simulink model "Lab4_DataLog_hw_solution"  (R2025b)
settings: Solver=FixedStepDiscrete  StartTime=0.0  StopTime=30  FixedStep=50e-6  RelTol=1e-3  EnableMultiTasking=on
undefined symbols (not defined in the file or in its folder): A0, A4, ADC, B0, C10, C11, C12, C13, C14, C15, C2, C3, C4, C5, CND4max, D0, D1, D10, D12, D13, D14, D2, D3, D4, D5, D6, D9, DiscIntNeverNeededParam, Max, MaxPer, ms, NumBits1, NumBits2, P1, P17, P20, P35, P36, P37, P38, P43, P44, P45, P46, P47, P48, P49, P50, P51, P52, P54, P55, P58, P59, P61, P62, P63, Pin, PWM1_Trg1, Resol ... (+2)
libraries: simulink x31, MCHP_Blockset x20
(part 1 of 5)
PreSaveFcn:
  | try, MCHP_Fun.syncToolchainOptions(gcs); catch, end  %MCHP_PRESAVE_SYNC_V1
Description:
  | v1.0 (2026-06-12): created template from Developpements dev model; added Title/HowTo root annotations + inner PINOUT (Pegasus pin map), fixed stale MaskType (CK256MP508->AK512MC510), SimulationMode external->normal.
  | v1.1 (2026-06-12): fancy annotation pass - coloured header band, spec badges, boxed callouts, keyboard-key HowTo, category-coloured PINOUT.
  | v1.1 (2026-06-12): fancy annotation pass - coloured header band, spec badges, boxed callouts, keyboard-key HowTo, category-coloured PINOUT.
  | v1.2 (2026-06-13): folded original detailed pinout into the new PINOUT (added System/Master/Compiler, PWM-config, UART-baud, Digital-I/O sections); removed superseded <!DOCTYPE> pinout (had M1_LED2=RA5 error) and old UART note; deduplicated PINOUT. Kept diagram-area section labels.
settings Model: SimulationMode=external  ExtModeEnableFloating=off  ExtModeTrigDuration=20  Creator=Lubin Kerhuel  LastModifiedBy=Lubin Kerhuel
settings SolverCC: AlgebraicLoopSolver=TrustRegion
settings OptimizationCC: DefaultUnderspecifiedDataType=single  EnhancedBackFolding=on  BooleansAsBitfields=on  PassReuseOutputArgsAs=Individual arguments  ZeroExternalMemoryAtStartup=off  ZeroInternalMemoryAtStartup=off  OptimizeBlockOrder=speed  DifferentSizesBufferReuse=on  EfficientTunableParamExpr=on
settings DebuggingCC: MultiTaskDSMMsg=none  MultiTaskCondExecSysMsg=none  MultiTaskRateTransMsg=warning  ParameterTunabilityLossMsg=error  ArithmeticOperatorsInVariantConditions=warning
settings HardwareCC: ProdBitPerPointer=32.0  ProdBitPerSizeT=32.0  ProdBitPerPtrDiffT=32.0  ProdLargestAtomicInteger=Long  ProdWordSize=32.0  ProdLongLongMode=on  ProdHWDeviceType=Generic->Custom
settings ModelReferenceCC: ModelReferenceNumInstancesAllowed=Single
settings SFSimCC: MATLABDynamicMemAlloc=off  CustomCodeUndefinedFunction=UseInterfaceOnly
settings RTWCC: SystemTargetFile=MCHP_dsPIC33A_noTMF_stf.tlc  TLCOptions="-aExtModeXCPClassicInterface=0  -aCreateExtModeTypes=1 -aExtModeXCPSimulationTimeInTicks=1"  TemplateMakefile=MCHP_dsPIC33A.tmf  Toolchain=MPLAB XC-DSC - v4.00 for dsPIC DSCs (Microchip)  BuildConfiguration=Specify  GPUComputeCapability=3.5  Description=Microchip Embedded Target dsPIC33A no TMF (real-time)
settings CodeAppCC: ForceParamTrailComments=on  IgnoreCustomStorageClasses=off  MaxIdLength=255.0  OperatorAnnotations=on  SimulinkDataObjDesc=on  SFDataObjDesc=on  InsertBlockDesc=on
settings STFCustomTargetCC: SystemTargetFile=MCHP_dsPIC33A_noTMF_stf.tlc  TargetLangStandard=C99 (ISO)  CodeReplacementLibrary=Microchip Code Replacement Library for dsPIC33A - (experimental)  MultiwordLength=256.0  ConcurrentExecutionCompliant=off  CombineOutputUpdateFcns=on  CombineSignalStateStructs=on  ERTCustomFileBanners=on  SubcomponentCodeInterfacePackaging=Nonreusable function  RemoveResetFunc=on  MATLABClassNameForMDSCustomization=Simulink.SoftwareTarget.ERTCustomization  GRTInterface=off  UseToolchainInfoCompliant=on  TIMER_PRESCALER="[-1 -1 -1  0  0 -1 -1 -1 -1 -1 -1 -1]"  GCC1=xc-dsc-gcc.exe  MCHP_MULTITHREAD_COMPILATION=on  LDFLAGS='--heap=1024,--report-mem,-Map=$(PRODUCT_NAME).map,-cref,-lq-dsp,--memorysummary,memoryfile.xml,--gc-sections'  ProduceHexOutput=off  MCHP_AUTO_FLASH=off  HOST_PLATFORM=PC  GCCPATH=C:/PROGRA~1/MICROC~1/xc-dsc/v4.00/bin  RTWGenSettings_txt="s.RefMasterBlk='Lab4_DataLog_hw_solution/BOARD MCLV-48V-300W dsPIC33AK512MC510 MC DIM1/Microchip Master';s.ChipIdN='[33  512  510]';s.ChipIdL1='AK';s.ChipIdL2='MC';s.ChipIdL3=' ';s.arch3='33A';s.ChipId='33AK512MC510';s.Arch='8';s.bitFieldsSFR='7';s.ChipRAM='32768';s.ChipRAM_XBegin='16384';s.ChipRAM_dma='[-1 -1]';s.AIVT_EN='0';s.FuseConfigTxt='#pragma config FICD_JTAGEN = OFF\\\\n#pragma config FWDT_WDTEN = SW\\\\n  ';s.TimeStep_Timer='-1';s.TimeStep_SyncADC='1';s.ADPCFG='0';s.ANSEL_Exist='1';s.ANSEL='[61439     -1  13287  40832      1     -1     -1     -1     -1     -1     -1]';s.TRIS='[65535  65535  65511  65520  65523  65533     -1     -1     -1     -1     -1     -1     -1     -1     -1     -1     -1     -1     -1     -1     -1     -1     -1     -1     -1     -1     -1     -1     -1     -1     -1     -1     -1     -1     -1     -1     -1     -1     -1     -1     -1     -1     -1     -1     -1     -1     -1     -1     -1     -1     -1     -1     -1     -1     -1     -1     -1]';s.RPOR='[-1         -1         -1         -1         -1         -1         -1         -1   83886080          6  352321536  318767104   33620995         -1         -1         -1         -1         -1         -1         -1         -1         -1         -1         -1         -1         -1         -1         -1         -1         -1         -1         -1         -1         -1         -1         -1]';s.RPINR='[-1       -1       -1       -1       -1       -1       -1       -1       -1    15935       -1       -1       -1  2818095       -1       -1       -1       -1       -1       -1       -1       -1       -1       -1       -1       -1       -1       -1]';s.LATSET='[-1 -1 -1 -1 -1 -1 -1 -1 -1 -1 -1 -1 -1 -1 -1 -1 -1 -1 -1 -1 -1 -1 -1 -1 -1 -1 -1 -1 -1 -1 -1 -1 -1 -1 -1 -1 -1 -1 -1 -1 -1 -1 -1 -1 -1 -1 -1 -1 -1 -1 -1 -1 -1 -1 -1 -1 -1]';s.LATCLR='[-1 -1 -1 -1 -1 -1 -1 -1 -1 -1 -1 -1 -1 -1 -1 -1 -1 -1 -1 -1 -1 -1 -1 -1 -1 -1 -1 -1 -1 -1 -1 -1 -1 -1 -1 -1 -1 -1 -1 -1 -1 -1 -1 -1 -1 -1 -1 -1 -1 -1 -1 -1 -1 -1 -1 -1 -1]';s.ODC='[-1 -1 -1 -1 -1 -1 -1 -1 -1 -1 -1 -1 -1 -1 -1 -1 -1 -1 -1 -1 -1 -1 -1 -1 -1 -1 -1 -1 -1 -1 -1 -1 -1 -1 -1 -1 -1 -1 -1 -1 -1 -1 -1 -1 -1 -1 -1 -1 -1 -1 -1 -1 -1 -1 -1 -1 -1]';s.CNPU='[-1 -1 -1 -1 -1 -1 -1 -1 -1 -1 -1 -1 -1 -1 -1 -1 -1 -1 -1 -1 -1 -1 -1 -1 -1 -1 -1 -1 -1 -1 -1 -1 -1 -1 -1 -1 -1 -1 -1 -1 -1 -1 -1 -1 -1 -1 -1 -1 -1 -1 -1 -1 -1 -1 -1 -1 -1]';s.CNPD='[-1 -1 -1 -1 -1 -1 -1 -1 -1 -1 -1 -1 -1 -1 -1 -1 -1 -1 -1 -1 -1 -1 -1 -1 -1 -1 -1 -1 -1 -1 -1 -1 -1 -1 -1 -1 -1 -1 -1 -1 -1 -1 -1 -1 -1 -1 -1 -1 -1 -1 -1 -1 -1 -1 -1 -1 -1]';s.PortConfigTxt=' ';s.CLKDIV='0';s.PLLFBD='-1';s.PLLDIV='16815713';s.QUARTZ='8000000';s.SWITCH_OSC='16386';s.PLLRNG='-1';s.MASTER_BusyFlag='-1';s.POWERSAVE='0';s.MIPS='200000000';s.FLASH_ECC='0';s.PBxDIV='[-1]';s.CLKx_INTDIV='[-1 -1 -1 -1  0  1  0  0  0 -1 -1  0  0]';s.CLKx_FRACDIV='[-1   -1   -1   -1    0  256    0    0    0   -1   -1    0    0]';s.AN_type2='1';s.ACLKCON_reg='-1';s.FRC_TUN_REG='0';s.BFRC_TUN_REG='0';s.nTIMERS='3';s.nSCCP='9';s.DOS_04094_cpu_33a_v1_dspic33a='1';s.DOS_04436_perseus_dspic33a='0';s.DOS_04928_gpio_ports_upb_v2_dspic33a='1';s.DOS_02672_math_progcrc_upb_v1_dspic33a='1';s.DOS_04993_sec_32bit_cp_upb_v1_dspic33a='1';s.DOS_03459_adc_pc_ctrl_upb_v2_dspic33a='0';s.DOS_04302_pwm_pc_upb_v3_dspic33a='0';s.DOS_03076_uart_protocol_upb_v1_dspic33a='1';s.DOS_01482_spi_i2s_upb_v1_dspic33a='1';s.DOS_05155_i2c_upb_v4_dspic33a='1';s.DOS_02359_sent_j2716_upb_v1_dspic33a='1';s.DOS_05177_qei_32b_upb_v2_dspic33a='1';s.DOS_01512_ccp_mccp_upb_v1_dspic33a='1';s.DOS_03496_dac_pdm_nbit_upb_v2_dspic33a='0';s.DOS_02673_tmr_classa_upb_v1_dspic33a='1';s.DOS_04776_perf_mon_upb_v1_dspic33a='1';s.DOS_03680_pfm_pbu_33a_upb_v1_dspic33a='1';s.DOS_04649_sec_pac_upb_v0_dspic33a='0';s.DOS_03966_io_integrity_monitor_upb_v1_dspic33a='1';s.DOS_04641_biss_master_upb_v1_dspic33a='1';s.DOS_04077_dma_upb_v1_dspic33a='1';s.DOS_04549_nvm_ctrl_32bit_upb_v1_dspic33a='1';s.DOS_04449_clk_cru_33a_upb_v1_dspic33a='1';s.DOS_03850_clk_monitor_upb_v1_dspic33a='1';s.DOS_04342_osc_rc8mhz_ctrl_upb_v4_dspic33a='1';s.DOS_04650_wdt_upb_v4_dspic33a='1';s.DOS_05178_ptg_pc_upb_v2_dspic33a='1';s.DOS_04181_data_ram_ctrl_upb_v1_dspic33a='1';s.DOS_04735_wdt_dmt_upb_v6_dspic33a='1';s.DOS_01577_cla_clc_upb_v1_dspic33a='1';s.DOS_03516_pwr_sib_upb_v3_dspic33a='0';s.DOS_03495_amp_pad_opamp_ctrl_upb_v2_dspic33a='1';s.DOS_02481_WACK_MC_Config='0';s.DOS_03088_pfm_cache_ocp_v2_WACK='0';s.DOS_02819_pfm_ctrl_32bit_upb_v2='0';s.DOS_02674_wdt_upb_v1_32bit='0';s.DOS_01520_wdt_dmt_upb_v1='0';s.DOS_02869_icd_jtag_bvci_upb_v2='0';s.DOS_02823_WACJ_clk_cru_upb_v2='0';s.DOS_02823_WACN_clk_cru_upb_v2='0';s.DOS_01423_RPINRx='0';s.DOS_02481_RPORx='0';s.DOS_02511_pwr_sib_upb_v1_32bit='0';s.DOS_02907_WACN_GP_int_evic_v3='0';s.DOS_01500_dma_bvci_v2='0';s.DOS_02141_tmr_classa_pb_v2='0';s.DOS_02815_tmr_classb_upb_v1='0';s.DOS_00740_icap_pb_v1='0';s.DOS_00749_ocmp_pb_v1='0';s.DOS_01441_i2c_upb_v1_32bit='0';s.DOS_01329_spi_pb_v2='0';s.DOS_02478_uart_irda_upb_v1_32bit='0';s.DOS_03554_cmp_control_upb_v2_32bit='0';s.DOS_01445_dac_nbit__control_upb_v1_32bit='0';s.DOS_01461_afe_ctmu_con_upb_v1='0';s.DOS_01577_cla_clc_upb_v1_32bit='0';s.DOS_02467_gpio_ports_upb_v1='0';s.DOS_02508_adc_sar_ctrl_upb_v1_PIC32MK='0';s.DOS_01261_tmr_rtcc_pb_v2='0';s.DOS_01475_lpwr_deep_sleep_ctrl_v2='0';s.DOS_EIP_00136_ssx_v1='0';s.DOS_02907_WACK_MC_int_evic_v3='0';s.DOS_02514_dfm_strl_sst_upb_v1='0';s.DOS_02472_ppi_pmp16_upb_v1='0';s.DOS_02813a_usb_otgcore_pb_v3='0';s.DOS_02481_WACP_Config='0';s.DOS_02907_WACP_int_evic_v3='0';s.DOS_01477_pwm_mc_upb_v1='0';s.DOS_01494_qei_32b_upb_v1='0';s.DOS_02508_WACP_adc_sar_ctrl_upb_v1='0';s.DOS_01261_tmr_rtcc_WACJ_K_N_P_pb_v2='0';s.DOS_02907_WACN_MC_int_evic_v3='0';s.DOS_03247_can_fd_upb_v2_pic32mk='0';s.DOS_02481_WACJ_MC_Config='0';s.DOS_02569_pfm_cache_ocp_v1='0';s.DOS_02481_WACJ_MC_int_evic_v3='0';s.DOS_01459_ptg_pc_upb_v1_SIC='0';s.DOS_01427_cmp_control_upb_v1_32bit='0';s.DOS_01152_can_bvci_v1='0';s.DOS_02787_WACD_Config='0';s.DOS_00800_dac_4bit_ctrl_pb_v1='0';s.DOS_01539_icd_jtag_pb_v2='0';s.DOS_02823_clk_cru_upb_v2='0';s.DOS_01423_RPORx='0';s.DOS_02907_WACD_int_evic_v3='0';s.DOS_00734_uart_irda_pb_v1='0';s.DOS_00687_tmr_classa_pb_v1='0';s.DOS_00745_tmr_classb_pb_v1='0';s.DOS_02508_adc_sar_ctrl_upb_v1='0';s.DOS_00866_cmp_control_pb_v2='0';s.DOS_01114_eth_bvci_v1='0';s.DOS_02831_usb_clk_rst_v2='0';s.DOS_01643_pfm_cache_ahb_v2='0';s.DOS_EIP_00206r5_sqi_v2='0';s.DOS_EIP_00124_usb_hs_otgcore_v1='0';s.DOS_EIP_00218_math_rng_ahbs_v2='0';s.DOS_EIP_00109_ebi_v1='0';s.DOS_EIP_00158_crypto_v1='0';s.DOS_05557_serpens_dspic33a='0';s.DOS_05972_adc_12b_upb_v3_adc_dspic33a='0';s.DOS_03681_bmx_33a_upb_v1_dspic33a='0';s.DOS_05226_pwm_pc_upb_v4_dspic33a='1';s.DOS_05514_qei_32b_upb_v3_dspic33a='0';s.DOS_02050_tmr_rtcc_upb_v1_dspic33a='0';s.DOS_05431_dac_pdm_nbit_upb_v3_dspic33a='1';s.DOS_04649_sec_pac_upb_serpens_dspic33a='0';s.DOS_05801_dma_upb_v2_dspic33a='0';s.DOS_05692_pwr_sib_upb_v5_dspic33a='0';s.DOS_05420_amp_vref_ctl_upb_v1_dspic33a='1';s.DOS_05346_sec_cam_v2_dspic33a='1';s.DOS_06006_adc_soft_code_seq_v2_adc_dspic33a='0';s.DOS_05442_icd_trace_33a_v1_dspic33a='0';s.DOS_04537_can_fd_upb_v3_dspic33a='1';s.DOS_05308_pegasus_dspic33a='1';s.DOS_02976_adc_12b_upb_v2_dspic33a='1';s.DOS_05404_adc_pc_ctrl_upb_v3_dspic33a='1';s.DOS_05226_apwm_pc_upb_v4_dspic33a='1';s.DOS_04649_sec_pac_upb_v1_dspic33a='1';s.DOS_05461_pwr_sib_upb_v4_dspic33a='1';s.DOS_03267_adc_soft_code_seq_v1_dspic33a='1';s.DOS_05830_blueRidge_dspic33a='0';s.DOS_05972_adc_12b_upb_v3_itc_dspic33a='0';s.DOS_05828_pfm_pbu_33a_upb_v2_dspic33a='0';s.DOS_05765_math_rdc_upb_v1_32bit='0';s.DOS_05908_math_cic_upb_v2_32bit='0';s.DOS_05592_pwr_monitor_sib_upb_v1='0';s.DOS_05924_bus_dual_die_upb_v2='0';s.DOS_06048_sec_cam_v3_dspic33a='0';s.DOS_05922_i3c_upb_v1_32bit='0';s.DOS_06006_adc_soft_code_seq_v2_dspic33a='0';s.DOS_02551_cpu_16bit_v7='0';s.DOS_01520_wdt_dmt_upb_v1_16bit='0';s.DOS_02359a_sent_j2716_upb_v1='0';s.DOS_02672_math_progcrc_upb_v1_16bit='0';s.DOS_01577_cla_clc_upb_v1='0';s.DOS_02915_ecc_v2='0';s.DOS_02673_tmr_classa_upb_v1_16bit='0';s.DOS_01494_qei_32b_upb_v1_16bit='0';s.DOS_01441_i2c_upb_v1_16bit_TLAH='0';s.DOS_03076_uart_protocol_upb_v1_16bit='0';s.DOS_01482='0';s.DOS_01483_pwm_16bit='0';s.DOS_04884_WAC0B='0';s.DOS_02316_nvm_ctrl_v1_16bit='0';s.DOS_03349_amp_pad_opamp_ctrl_upb_v1='0';s.DOS_02653_afe_current_bias_ctrl_upb_v1_16bit='0';s.DOS_01459_ptg_pc_upb_v1_16bit='0';s.DOS_01512_ccp_mccp_upb_v1_16bit='0';s.DOS_02519_dma_sfr_16bit_v2='0';s.DOS_02508c11='0';s.DOS_02475_dac_pdm_nbit_upb_v1_16bit='0';s.DOS_02467_gpio_upb_v1_16bit='0';s.DOS_00805_rst_integration_v4='0';s.DOS_02659_clk_sib_v12='0';s.DOS_02237_osc_dco_ctrl_upb_v1_16bit='0';s.DOS_02674_wdt_upb_v1_16bit='0';s.DOS_01407='0';s.DOS_03247_CAN_FD_UPB_V2_16_bit='0';s.DOS_03994_WAC07='0';s.DOS_02472_ppi_pmp16_upb_v1_16bit='0';s.DOS_02949_WACG='0';s.DOS_02552_msi_upb_v1_Master='0';s.DOS_03667_pwm_pc_upb_v2_16bit='0';s.DOS_04180_drm_ctrl_ecc_v1='0';s.DOS_03431_STX03='0';s.DOS_03516_pwr_sib_upb_v3='0';s.DOS_02552_msi_upb_v1_Slave='0';s.DOS_04621_amp_pga_ctrl_upb_v3='0';s.DOS_02497_WACV='0';s.DOS_02593_amp_pga_ctrl_pb_v2_16bit='0';s.DOS_03029_WACH='0';s.DOS_01483_apwm_16bit='0';s.DOS_04797_WAC0A='0';s.DOS_04797_WAC09='0';s.DOS_03662_WACU='0';s.DOS_00794='0';s.DOS_00931='0';s.DOS_00932='0';s.DOS_00942='0';s.DOS_00938='0';s.DOS_00996='0';s.DOS_00997='0';s.DOS_00998='0';s.DOS_00209='0';s.DOS_01555_adc='0';s.DOS_01293='0';s.DOS_00828='0';s.DOS_01116='0';s.DOS_01017_RPORx='0';s.DOS_01017_RPINRx='0';s.DOS_01555_nvm_tsmc18_v2_16bit='0';s.DOS_00804='0';s.DOS_00826='0';s.DOS_01555_TLAK_PMDx='0';s.DOS_01555_TLAK_INT_='0';s.DOS_00933='0';s.DOS_01555='0';s.DOS_01555_ptg='0';s.DOS_00929='0';s.DOS_00958='0';s.DOS_01117_PORTx='0';s.DOS_00999='0';s.DOS_01198='0';s.DOS_01041='0';s.DOS_00892='0';s.DOS_01287_TLAC_PMDx='0';s.DOS_01287_TLAC_INT_='0';s.DOS_01424='0';s.DOS_01332='0';s.DOS_01113='0';s.DOS_01017_PMDx='0';s.DOS_00927='0';s.DOS_01080='0';s.DOS_01468_PMBA_current_source='0';s.DOS_02291_PGA='0';s.DOS_01467_Comparator='0';s.DOS_01498_TLAY='0';s.DOS_00993_PLL_120MHz='0';s.DOS_01332_ptg_pc_v1='0';s.DOS_00958_pwm_TLAY='0';s.TLAY_IOPorts='0';s.DOS_00929q='0';s.DOS_02415_spi_v5='0';s.DOS_RPINRx_16bit_2='0';s.DOS_01497_TLAH_PMDx='0';s.DOS_02550_TLAL_INT='0';s.DOS_00958_pwm_TLAH='0';s.DOS_01287_TLAH_INT_='0';s.DOS_00794_cpu_16bit_v3='0';s.DOS_02192_TLCD_PMDx='0';s.DOS_02192_TLCD_INT_='0';s.DOS_02192_cmp='0';s.DOS_00958_pwm_TLCD='0';s.DOS_02192_PORTx_TLCD='0';s.DOS_00936='0';s.DOS_00995='0';s.DOS_00546='0';s.DOS_00474='0';s.UART_TX_IMPLEMENTATION='[5  5]';s.UART_RX_IMPLEMENTATION='[6  6]';s.UART_TX_DMACHANNEL='[0  1]';s.UART_HALF_DUPLEX_MODE='[0  0]';s.UART_TX_THREAD_PROTECTION='[9  9]';"  TIMER_START="[0  0  0  1  0]"  OPTIM_GCC=-O3 -mno-eds-warn -mconst-in-data -mlarge-code -mlarge-data -mlarge-scalar -g -Wa,--reorder -ffunction-sections -fdata-sections  TIMER_WIDTH="[16  16  16  32  16  16  16  16  16  16  16  16]"  MCHP_CompiledTime_ModelSampleTimes_Txt=s(1).Value=reshape([0 0],1,2);s(1).Description='Continuous';s(1).ColorRGBValue=reshape([0 0 0],1,3);s(1).Annotation='Cont';s(1).TID=0;s(1).Owner=[];s(1).ComponentSampleTimes=[];s(2).Value=reshape([5e-05 0],1,2);s(2).Description='Discrete 1';s(2).ColorRGBValue=reshape(MCHP_Fun.Hex2num('[3FCF1F1F1F1F1F1F 3FC3131313131313 3FE5151515151515]'),1,3);s(2).Annotation='D1';s(2).TID=1;s(2).Owner=[];s(2).ComponentSampleTimes=[];s(3).Value=reshape([0.0001 0],1,2);s(3).Description='Discrete 2';s(3).ColorRGBValue=reshape(MCHP_Fun.Hex2num('[3FD0D0D0D0D0D0D1 3FD9D9D9D9D9D9DA 3FEFBFBFBFBFBFC0]'),1,3);s(3).Annotation='D2';s(3).TID=2;s(3).Owner=[];s(3).ComponentSampleTimes=[];s(4).Value=reshape([0.0005 0],1,2);s(4).Description='Discrete 3';s(4).ColorRGBValue=reshape(MCHP_Fun.Hex2num('[3FBC1C1C1C1C1C1C 3FE5555555555555 3FEBFBFBFBFBFBFC]'),1,3);s(4).Annotation='D3';s(4).TID=3;s(4).Owner=[];s(4).ComponentSampleTimes=[];s(5).Value=reshape([0.001 0],1,2);s(5).Description='Discrete 4';s(5).ColorRGBValue=reshape(MCHP_Fun.Hex2num('[3FD2121212121212 3FE9797979797979 3FE0D0D0D0D0D0D1]'),1,3);s(5).Annotation='D4';s(5).TID=4;s(5).Owner=[];s(5).ComponentSampleTimes=[];s(6).Value=reshape([0.01 0],1,2);s(6).Description='Discrete 5';s(6).ColorRGBValue=reshape(MCHP_Fun.Hex2num('[3FED5D5D5D5D5D5D 3FE7575757575757 3FC8181818181818]'),1,3);s(6).Annotation='D5';s(6).TID=5;s(6).Owner=[];s(6).ComponentSampleTimes=[];s(7).Value=reshape([0.1 0],1,2);s(7).Description='Discrete 6';s(7).ColorRGBValue=reshape(MCHP_Fun.Hex2num('[3FEF3F3F3F3F3F3F 3FEF7F7F7F7F7F7F 3FB5151515151515]'),1,3);s(7).Annotation='D6';s(7).TID=6;s(7).Owner=[];s(7).ComponentSampleTimes=[];s(8).Value=reshape([-1 -2],1,2);s(8).Description='Asynchronous 1';s(8).ColorRGBValue=reshape(MCHP_Fun.Hex2num('[3FE8181818181818 3FD7171717171717 3FEF7F7F7F7F7F7F]'),1,3);s(8).Annotation='A1';s(8).TID=7;s(8).Owner={ 'MCHP_MCLV48V300W_dsPIC33AK512MC510_DIM_HallSensors_DataLog/Interrupt'};s(8).ComponentSampleTimes=[];s(9).Value=reshape([Inf Inf],1,2);s(9).Description='Constant';s(9).ColorRGBValue=reshape(MCHP_Fun.Hex2num('[3FEA3A3A3A3A3A3A 3F90101010101010 3FE1717171717171]'),1,3);s(9).Annotation='Inf';s(9).TID=-2;s(9).Owner=[];s(9).ComponentSampleTimes=[];s(10).Value=[];s(10).Description='Multirate';s(10).ColorRGBValue=reshape(MCHP_Fun.Hex2num('[3FE1717171717171 3FD999999999999A 3F98181818181818]'),1,3);s(10).Annotation='M';s(10).TID=[];s(10).Owner=[];s(10).ComponentSampleTimes=[];  BIN2HEX=xc-dsc-bin2hex  TIMER_PERIOD="[0          0          0  199999999      65535]"  LINKER_SCRIPT=p33AK512MC510.gld  EXTMODE_DATA_UPLOAD=on  MCHP_XCP_MemoryBlockParameters=[10 10]  AssemblyListing=off  OBJDUMP=xc-dsc-objdump  AR1=xc-dsc-ar  LinkWithMaster=off  PIC_REF=33AK512MC510
settings ERTTargetCC: ExtMode=on  ExtModeTransport=1.0  ExtModeStaticAlloc=on  ExtModeStaticAllocSize=2048.0  ExtModeMexFile=ext_xcp  ExtModeMexArgs=1 34 8000000 './MCHP_MCLV48V300W_dsPIC33AK512MC510_DIM_HallSensors_DataLog.X/MCHP_MCLV48V300W_dsPIC33AK512MC510_DIM_HallSensors_DataLog.elf'  ExtModeIntrfLevel=Level2 - Open  InlinedParameterPlacement=Hierarchical  ERTSrcFileBannerTemplate=MCHP_dsPIC_code_template.cgt  ERTHdrFileBannerTemplate=MCHP_dsPIC_code_template.cgt  ERTDataSrcFileTemplate=MCHP_dsPIC_code_template.cgt  ERTDataHdrFileTemplate=MCHP_dsPIC_code_template.cgt  ERTCustomFileTemplate=MCHP_main.tlc  MaxLineWidth=110.0  DynamicArrayContainerType=coder::array  TargetLangStandard=C99 (ISO)  CodeReplacementLibrary=Microchip Code Replacement Library for dsPIC33A - (experimental)  ParMdlRefBuildCompliant=off  CompOptLevelCompliant=off  ConcurrentExecutionCompliant=off  CombineSignalStateStructs=on  SubcomponentCodeInterfacePackaging=Nonreusable function  SupportContinuousTime=on  SupportNonInlinedSFcns=on  ModelStepFunctionPrototypeControlCompliant=off  CPPClassGenCompliant=off

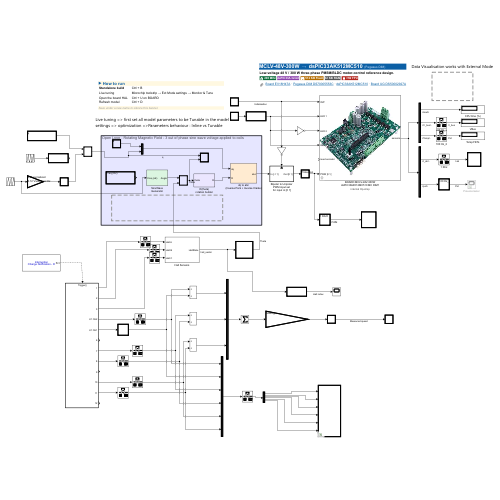
[thumbnail: Simulink's stored preview of the top-level diagram]
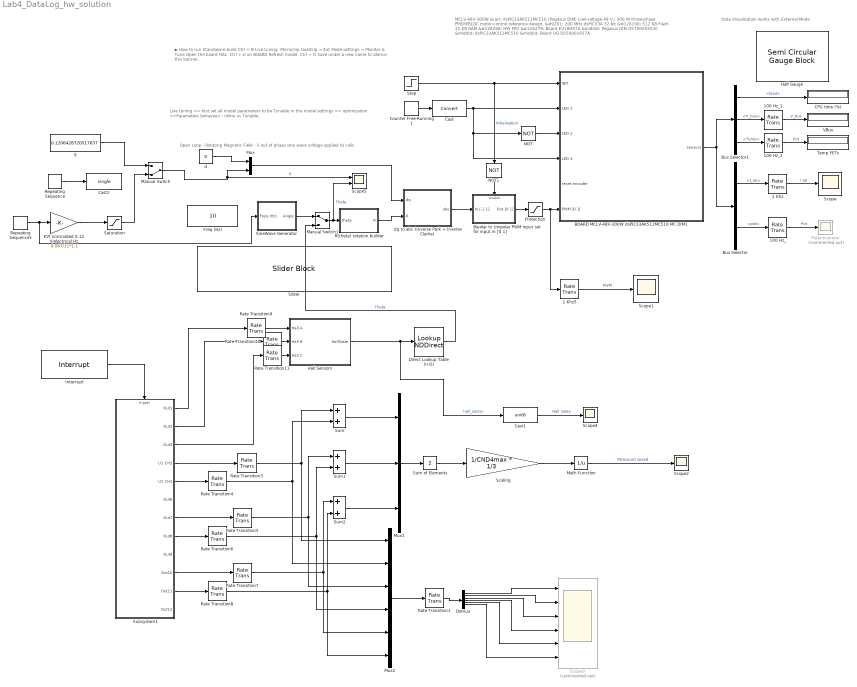
== system Lab4_DataLog_hw_solution ==
  note: Data Visualisation works with External Mode
  note: Open Loop - Rotating Magnetic Field - 3 out of phase sine wave voltage applied to coils
  note: MCLV-48V-300W &rarr; dsPIC33AK512MC510 (Pegasus DIM)
      | Low-voltage 48 V / 300 W three-phase PMSM/BLDC motor-control reference design.
      | &#9201; 200 MHz dsPIC33A 32-bit &#128190; 512 KB Flash 32 KB RAM &#128268; HW FPU
      | &#128279; Board EV18H47A &middot; Pegasus DIM DS70005553C &middot; dsPIC33AK512MC510 &middot; Board UG DS50002927A
  note: ▶ How to run
      | Standalone build
      |
      | Ctrl + B
      |
      | Live tuning
      | ​
      | Microchip toolstrip → Ext Mode settings → Monitor & Tune
      |
      | Open the board HAL
      | ​
      | Ctrl + U on BOARD
      |
      | Refresh model
      | ​
      | Ctrl + D
      |
      | Save under a new name to silence this banner.
  note: Live tuning => first set all model parameters to be Tunable in the model settings => optimization =>Parameters behaviour : Inline vs Tunable
  1 Khz : RateTransition  Deterministic=off  OutPortSampleTime=50e-6
  1 Khz5 : RateTransition  Deterministic=off  OutPortSampleTime=.001
  100 Hz_ : RateTransition  Deterministic=off  OutPortSampleTime=.01
  100 Hz_1 : RateTransition  Deterministic=off  OutPortSampleTime=.01
  100 Hz_2 : RateTransition  Deterministic=off  OutPortSampleTime=.01
  BOARD MCLV-48V-300W dsPIC33AK512MC510 MC DIM1 : Subsystem  mask(MCLV-48V-300W - dsPIC33AK512MC510 MC DIM){boardVariants=internal Op-Amp, n=4, QEIResolution=1000, QEI_Reset=on logical input (software), QEI_Offset_settings=0, QEIOffset=0}
      mask prompts: boardVariants "board variants"; n "Motor poles pairs"; QEIResolution "Optical encoder resolution per mechanical rotation (lines)"; QEI_Reset "Optical encoder reset"; QEI_Offset_settings "Optical encoder offset (mechanical in rad)"; QEIOffset "Optical encoder offset (mechanical in rad)"
      mask help:
      | Template for motor control algorithm. Open subsystem (ctrl-u) for further customisation.
      |
      | Block bus output provices:
      |   - Current phase ia & ib, DC bus and potentiometer position
      |   - Buttons (0 when pressed, 1 for Btn 3 unconnected)
      |   - QEI position and velocity
      |   - MCU load and overload
      |
      | Block inputs:
      |   - INIT signal average the current phase ia and ib to be removed
      |   - LEDs
      |   - Reset encoder allows to align the motor while reseting the encoder
      |   - PWM normalized duty cycle value
      |
      | Model 50us base rate (20kHz) is synchronized with ADC conversion which is synchronized with the 50us PWM periods
      mask init:
      | BlksQEI = find_system(gcb,'FollowLinks','on','LookUnderMasks','all','ReferenceBlock','MCHP_Blockset/QEI/QEI');
      | QEI_Reset = get_param(gcb,'QEI_Reset');
      | if numel(BlksQEI) >= 1
      |     switch QEI_Reset
      |         case 'on index signal'
      |             set_param(BlksQEI{1},'PIMOD_mode','RESET position on each INDEX event');
      |         case 'on logical input (software)'        
      |             set_param(BlksQEI{1},'PIMOD_mode','position is cyclique between user defined boundaries'); 
      |         case 'custom setting'
      |             % do nothing 
      |     end
      | end % if
      | 
      |     BlksOpAmp = find_system(gcb,'FollowLinks','on','IncludeCommented','on','LookUnderMasks','all','ReferenceBlock','MCHP_Blockset/Analog IO/Op-Amp');
      |     if numel(BlksOpAmp) >= 1
      |         boardVariants = get_param(gcb,'boardVariants');
      |         switch boardVariants
      |             case 'internal Op-Amp'
      |                 set_param(BlksOpAmp{1},'Commented','off');
      |             case 'external Op-Amp'
      |                 set_param(BlksOpAmp{1},'Commented','on');
      |         end
      |     end % if
      settings: AttributesFormatString=%<boardVariants>
      mask TypeOptions boardVariants: internal Op-Amp | external Op-Amp
      mask TypeOptions n: 1 | 2 | 3 | 4 | 5 | 6 | 7 | 8 | 9 | 10 | 11 | 12 | 13 | 14 | 15 | 16
      mask TypeOptions QEI_Reset: on index signal | on logical input (software) | custom setting
      mask Callback QEI_Reset:
      | QEI_Reset = get_param(gcb,'QEI_Reset');
      | switch QEI_Reset
      |     case 'on index signal'
      |         QEIOffset = MCHP_Fun.Evalin('base','QEIOffset');
      |         set_param(gcb,'QEIOffset',num2str(QEIOffset));
      |         set_param(gcb,'MaskVisibilities',{'on';'on';'on';'on';'on';'off'});
      |     case 'on logical input (software)'
      |         set_param(gcb,'QEIOffset','0');
      |         set_param(gcb,'MaskVisibilities',{'on';'on';'on';'on';'off';'off'});
      |     case 'custom setting'
      |         set_param(gcb,'MaskVisibilities',{'on';'on';'on';'on';'on';'off'});
      |         % do nothing
      | end
      mask DialogControl n Tooltip: Number of pole pairs of the motor
      mask DialogControl QEIResolution Tooltip: encoder resolution per mechanical rotation
      mask DialogControl QEI_Reset Tooltip: enable encoder index signal if available. Otherwise align motor by applying a tension and set the rst input to 1
      mask DialogControl QEI_Offset_settings Tooltip: offset angle between encoder index and motor winding reference axis applied on theta_m and theta_e
      mask Display: image('MCHP_i_Board_MCLV_300W48V_reduced.jpg','center');
  Bipolar to Unipolar PWM input set for input in [0 1] : Subsystem
  Bus Selector : BusSelector  OutputSignals=ADC.I_ab,ADC.pot
  Bus Selector1 : BusSelector  OutputSignals=MCU.load,ADC.V_bus,Temp
  CPU time (%) : Display
  Cast : DataTypeConversion  SaturateOnIntegerOverflow=off  RndMeth=Floor
  Cast1 : DataTypeConversion  OutDataTypeStr=uint8  SaturateOnIntegerOverflow=off  RndMeth=Floor
  Cast2 : DataTypeConversion  OutDataTypeStr=single  SaturateOnIntegerOverflow=off  RndMeth=Floor
  Counter Free-Running1 : simulink/Sources/Counter Free-Running  NumBits=1  tsamp=0.1
  Demux : Demux  Outputs=6
  Direct Lookup Table (n-D) : LookupNDDirect  NumberOfTableDimensions=1  Table=[0 5 3 4 1 0 2 0 ] * pi/3  RemoveProtectionInput=on  TableDataTypeStr=single
  Freq (Hz) : Constant  Value=10  OutDataTypeStr=fixdt(1,32,10)  SampleTime=.1
  Half Gauge : SemiCircularGaugeBlock  FontColor=[0.0, 0.0, 0.0]
  Hall Sensors : Subsystem
  Interrupt : MCHP_Blockset/System Functions/Interrupt  Interruption_TXT=CND  InterruptionLongDesc=Change Notification - D  IntPriority=5  IntPriority_Info=Priority 5 (set by MCHP_MCLV48V300W_dsPIC33AK512MC510_DIM_HallSensors_DataLog/Subsystem1/Change Notification1)  StartupExecute=off  ClearActionState=CND:if:CNDIF:0=1  Status=OK  MCHP_MASTERLINK=Lab4_DataLog_hw_solution/BOARD MCLV-48V-300W dsPIC33AK512MC510 MC DIM1/Microchip Master  FPUNoSave=on  Triggered_Sub_TimeSource=is derived from model base rate  TrigsPeriod=0  TIMER_Resolution_TXT="Resol: 0.01(us)  -  MaxPer: 0.655(ms)"  Info=0  SS_ASYNCHRONOUS_INTERRUPT=1  SS_TIMESOURCE=1  SS_AsyncTimerRes=-1  SS_AsyncTaskPriority=5  SS_ARCH=16
      settings: SourceProductName=MPLAB Device Blocks for Simulink
  KVf normalized 0.12 V/electrical Hz : Gain  Gain=0.067/11*1.1  OutDataTypeStr=single
  Manual Switch : ManualSwitch  CurrentSetting=0
  Manual Switch1 : ManualSwitch
  Math Function : Math  Operator=reciprocal  OutDataTypeStr=single
  Mux : Mux  Inputs=2
  Mux1 : Mux  Inputs=3
  Mux2 : Mux  Inputs=6
  NOT : Logic  Operator=NOT  IconShape=distinctive  AllPortsSameDT=off  OutDataTypeStr=boolean
  NOT1 : Logic  Operator=NOT  IconShape=distinctive  AllPortsSameDT=off  OutDataTypeStr=boolean
  Potentiometer : Scope  Commented=on
      settings: ActiveDisplayYMinimum=0.51865  ActiveDisplayYMaximum=0.52073
  Protection : Saturate  UpperLimit=1  LowerLimit=0
  R(theta) rotation builder : Subsystem
  Rate Transition1 : RateTransition  Deterministic=off  OutPortSampleTime=1e-3
  Rate Transition{3,9..11} (4 alike) : RateTransition  Deterministic=off  OutPortSampleTime=50e-6
  Rate Transition{4..8} (5 alike) : RateTransition  Deterministic=off
  Repeating Sequence : simulink/Sources/Repeating Sequence  rep_seq_t=[0 1 2 4 5 6 15 20 30 ]  rep_seq_y=single([0 0 0.05 0.05 0.1 0.1 0.5 0.9 0])
  Repeating Sequence1 : simulink/Sources/Repeating Sequence  rep_seq_t=[0 1 20 30 ]  rep_seq_y=single([0 0 50 0])
  Saturation : Saturate  UpperLimit=0.95  LowerLimit=0.05
  Scaling : Gain  Gain=1/CND4max * 1/3  OutDataTypeStr=single
  Scope{,1..2,4} (4 alike) : Scope
      Scope settings: ActiveDisplayYMinimum=-25.669371587753297  ActiveDisplayYMaximum=10.583344289779664
      Scope1 settings: ActiveDisplayYMinimum=-0.71791580552235224  ActiveDisplayYMaximum=7.0575379566289485  DataLoggingVariableName=ScopeData3
      Scope2 settings: ActiveDisplayYMinimum=-0.91511729732155778  ActiveDisplayYMaximum=11.258249286562204  DataLoggingVariableName=ScopeData2
      Scope4 settings: ActiveDisplayYMinimum=-3.5201060827821484  ActiveDisplayYMaximum=32.450067600235343  DataLoggingVariableName=ScopeData5
  Scope3 : Scope  Commented=on  NumInputPorts=6
      settings: DataLoggingVariableName=ScopeData4
  Scope5 : Scope  NumInputPorts=2
      settings: ActiveDisplayYMinimum=-3.5201060827821484  ActiveDisplayYMaximum=32.450067600235343  DataLoggingVariableName=ScopeData6
  SineWave Generator : Subsystem
  Slider : SliderBlock  ScaleMax=1
  Step : Step  Before=1  After=0  SampleTime=0.1
  Subsystem1 : Subsystem
  Sum : Sum  SaturateOnIntegerOverflow=on
  Sum of Elements : Sum  Inputs=+
  Sum1 : Sum  SaturateOnIntegerOverflow=on
  Sum2 : Sum  SaturateOnIntegerOverflow=on
  Temp FETs : Display
  VBus : Display
  d : Constant  Value=0  OutDataTypeStr=single
  dq to abc (Inverse Park + Inverse Clarke) : Subsystem
  q : Constant  Value=0.1206428720517637  OutDataTypeStr=single
  wires:
  BOARD MCLV-48V-300W dsPIC33AK512MC510 MC DIM1/1(sensors) -> Bus Selector1/1, Bus Selector/1
  Bus Selector/1 -> 1 Khz/1  "<I_ab>"
  Bus Selector/2 -> 100 Hz_/1  "<pot>"
  1 Khz/1 -> Scope/1  "I ab"
  100 Hz_/1 -> Potentiometer/1  "Pot"
  Step/1 -> NOT1/1, BOARD MCLV-48V-300W dsPIC33AK512MC510 MC DIM1/1(INIT)  "Initialisation"
  Counter Free-Running1/1 -> Cast/1
  Cast/1 -> NOT/1, BOARD MCLV-48V-300W dsPIC33AK512MC510 MC DIM1/4(LED 3), BOARD MCLV-48V-300W dsPIC33AK512MC510 MC DIM1/2(LED 1)
  Mux/1 -> dq to abc (Inverse Park + Inverse Clarke)/1(dq)
  Bus Selector1/1 -> CPU time (%)/1  "<load>"
  Bipolar to Unipolar PWM input set for input in [0 1]/1(Out [0 1]) -> Protection/1
  NOT/1 -> BOARD MCLV-48V-300W dsPIC33AK512MC510 MC DIM1/3(LED 2)
  NOT1/1 -> Bipolar to Unipolar PWM input set for input in [0 1]/Enable
  dq to abc (Inverse Park + Inverse Clarke)/1(abc) -> Bipolar to Unipolar PWM input set for input in [0 1]/1(In [-1 1])
  Bus Selector1/2 -> 100 Hz_1/1  "<V_bus>"
  Bus Selector1/3 -> 100 Hz_2/1  "<Temp>"
  R(theta) rotation builder/1(R) -> dq to abc (Inverse Park + Inverse Clarke)/2(R)
  100 Hz_1/1 -> VBus/1  "V_bus"
  100 Hz_2/1 -> Temp FETs/1  "Pot"
  1 Khz5/1 -> Scope1/1  "PWM"
  Hall Sensors/1(HallState) -> Cast1/1, Direct Lookup Table (n-D)/1  "hall_sector"
  Protection/1 -> 1 Khz5/1, BOARD MCLV-48V-300W dsPIC33AK512MC510 MC DIM1/6(PWM ]0 1[)
  Direct Lookup Table (n-D)/1 -> Manual Switch1/2  "Theta"
  d/1 -> Mux/1
  Repeating Sequence/1 -> Cast2/1
  Sum2/1 -> Mux1/3
  Sum1/1 -> Mux1/2
  Sum/1 -> Mux1/1
  Mux1/1 -> Sum of Elements/1
  Scaling/1 -> Math Function/1
  Math Function/1 -> Scope2/1  "Measured speed"
  Mux2/1 -> Rate Transition1/1
  Rate Transition1/1 -> Demux/1
  Demux/1 -> Scope3/1
  Demux/2 -> Scope3/2
  Demux/3 -> Scope3/3
  Demux/4 -> Scope3/4
  Demux/5 -> Scope3/5
  Demux/6 -> Scope3/6
  Subsystem1/10(Out10) -> Rate Transition7/1
  Subsystem1/5(U1 CH1) -> Rate Transition4/1
  Subsystem1/4(U1 CH2) -> Rate Transition3/1
  Subsystem1/11(Out11) -> Rate Transition8/1
  Subsystem1/8(Out8) -> Rate Transition6/1
  Subsystem1/7(Out7) -> Rate Transition5/1
  Subsystem1/1(Out1) -> Rate Transition9/1
  Subsystem1/2(Out2) -> Rate Transition10/1
  Subsystem1/3(Out3) -> Rate Transition11/1
  Interrupt/1 -> Subsystem1/Trigger
  Rate Transition3/1 -> Sum/1, Mux2/1
  Rate Transition4/1 -> Sum/2, Mux2/2
  Rate Transition5/1 -> Sum1/1, Mux2/3
  Rate Transition6/1 -> Sum1/2, Mux2/4
  Rate Transition7/1 -> Sum2/1, Mux2/5
  Rate Transition8/1 -> Sum2/2, Mux2/6
  Rate Transition9/1 -> Hall Sensors/1(Hall A)
  Rate Transition10/1 -> Hall Sensors/2(Hall B)
  Rate Transition11/1 -> Hall Sensors/3(Hall C)
  Sum of Elements/1 -> Scaling/1
  Cast1/1 -> Scope4/1  "Hall index"
  Manual Switch/1 -> Scope5/1, Mux/2  "q"
  q/1 -> Manual Switch/1
  Manual Switch1/1 -> Scope5/2, R(theta) rotation builder/1(theta)  "Theta"
  SineWave Generator/1(Angle) -> Manual Switch1/1
  Repeating Sequence1/1 -> SineWave Generator/1(Freq (Hz)), KVf normalized 0.12 V/electrical Hz/1
  KVf normalized 0.12 V/electrical Hz/1 -> Saturation/1
  Saturation/1 -> Manual Switch/2
